simulink model "iotwifi"  (R2018b)
settings: Solver=FixedStepDiscrete  StartTime=0.0  StopTime=inf  RelTol=1e-3  EnableMultiTasking=on
undefined symbols (not defined in the file): Fi, Wi
libraries: arduinolib x1, arduinowifilib x1
settings Model: SimulationMode=external  ExtModeTrigDuration=2  Creator=grvbh  LastModifiedBy=grvbh
settings OptimizationCC: EnhancedBackFolding=on  PassReuseOutputArgsAs=Individual arguments  MaxStackSize=64  OptimizeBlockOrder=speed  DifferentSizesBufferReuse=on  OptimizationCustomize=off
settings DebuggingCC: ParameterPrecisionLossMsg=none  ParameterTunabilityLossMsg=error
settings HardwareCC: ProdBitPerInt=16  ProdBitPerPointer=16  ProdBitPerSizeT=16  ProdBitPerPtrDiffT=16  ProdLargestAtomicFloat=None  ProdWordSize=8  ProdHWDeviceType=Atmel->AVR  UseEmbeddedCoderFeatures=off  UseSimulinkCoderFeatures=off
settings SFSimCC: MATLABDynamicMemAlloc=off
settings RTWCC: SystemTargetFile=ert.tlc  HardwareBoard=Arduino Mega 2560  TemplateMakefile=ert_default_tmf  GenerateReport=on  Toolchain=Arduino AVR  BuildConfiguration=Faster Runs  IncludeHyperlinkInReport=on  LaunchReport=on  GenerateTraceInfo=on  GenerateTraceReport=on  GenerateTraceReportSl=on  GenerateTraceReportSf=on  GenerateTraceReportEml=on
settings CodeAppCC: ForceParamTrailComments=on  IgnoreCustomStorageClasses=off  OperatorAnnotations=on  SimulinkDataObjDesc=on  SFDataObjDesc=on  InsertBlockDesc=on
settings ERTTargetCC: SupportContinuousTime=on  SupportNonInlinedSFcns=on  SupportVariableSizeSignals=on

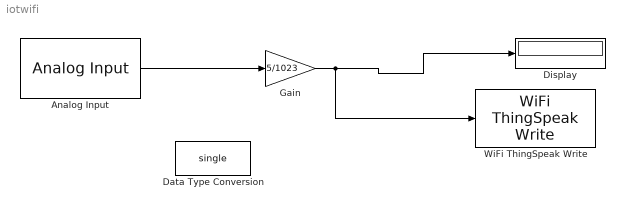
== system iotwifi ==
  Analog Input : arduinolib/Analog Input  pinNumber=1  ReadResultsOnly=off  ConversionTriggerSource=Software  ExternalTriggerType=uint32(0)  OutputDataType=uint16  EnableConversionCompleteNotify=off  EnableOuputStatus=off  SampleTime=1  blockPlatform=arduino
  Data Type Conversion : DataTypeConversion  OutDataTypeStr=single
  Display : Display
  Gain : Gain  Gain=5/1023  ParamDataTypeStr=single
  WiFi ThingSpeak Write : arduinowifilib/WiFi ThingSpeak Write  ChannelID_=725846  WriteAPIKey_=<FCHZ8VMHZZTW9XTU>  NumberOfFields=1  UpdateInterval_=60  PrintDiagnosticMessages_=off  LocationEnabled=off  LocationSource=Block dialog  blockPlatform=arduino  Interfacetype_=Wi-Fi  UpdateURL=0  StatusMessage=0  StatusEnabled=on  StatusSource=<empty>
      settings: SourceProductName=Simulink Support Package for Arduino Hardware  SourceProductBaseCode=ARDUINO
  wires:
  Analog Input/1 -> Gain/1
  Gain/1 -> WiFi ThingSpeak Write/1, Display/1
